simulink library "DABLib"  (R2016b)
settings: Solver=VariableStepAuto  StartTime=0.0  StopTime=10.0  RelTol=1e-3
undefined symbols (not defined in the file or in its folder): ln, sgn
libraries: DABLib x53, simulink_extras x2, simulink x1
(part 2 of 3)

== system DABLib/DABLibUtil/Medium evaporation fault f7 ==
  note: try from 0.3
  note: Fault  7
      | Medium evaporation or
      | critical pressure fault
  T[C] : Inport
  f7<0,1> : Inport  Port=2
  " " : Fcn  Expr=u(1)+200*u(4)+u(2)*u(3)*100
  Fault range <0..1> : Constant  Value=1.0
  "Fault streght saturation 0..100% " : Saturate  UpperLimit=1  LowerLimit=0
  "Fault threshold " : Constant  Value=0
  Mux4 : Mux
  Relational Operator1 : RelationalOperator  Operator=>  RndMeth=Nearest  InputSameDT=on
  Temperature range 0..300C : Saturate  UpperLimit=300  LowerLimit=0
  "Temperature range limiter 0..200C " : Saturate  UpperLimit=200  LowerLimit=0
  Tf[C] : Outport
  wires:
  " "/1 -> Temperature range 0..300C/1
  Relational Operator1/1 -> Mux4/4
  Mux4/1 -> " "/1
  "Fault streght saturation 0..100% "/1 -> Mux4/3, Relational Operator1/1
  "Fault threshold "/1 -> Relational Operator1/2
  Temperature range 0..300C/1 -> Tf[C]/1
  "Temperature range limiter 0..200C "/1 -> Mux4/1
  T[C]/1 -> "Temperature range limiter 0..200C "/1
  Fault range <0..1>/1 -> Mux4/2
  f7<0,1>/1 -> "Fault streght saturation 0..100% "/1

== system DABLib/DABLibUtil/NFSel ==
  f : Inport
  Constant4 : Constant  Value=FSel
  Constant5 : Constant  Value=0
  Demux : Demux  Outputs=19
  Multiport Switch : MultiPortSwitch  Inputs=20  SaturateOnIntegerOverflow=on  InputSameDT=on
  f(i) : Outport  InitialOutput=0
  wires:
  Demux/1 -> Multiport Switch/2
  Demux/2 -> Multiport Switch/3
  Demux/3 -> Multiport Switch/4
  Demux/4 -> Multiport Switch/5
  Demux/5 -> Multiport Switch/6
  Demux/6 -> Multiport Switch/7
  Demux/7 -> Multiport Switch/8
  Demux/8 -> Multiport Switch/9
  Demux/9 -> Multiport Switch/10
  Demux/10 -> Multiport Switch/11
  Demux/11 -> Multiport Switch/12
  Demux/12 -> Multiport Switch/13
  Demux/13 -> Multiport Switch/14
  Demux/14 -> Multiport Switch/15
  Demux/15 -> Multiport Switch/16
  Demux/16 -> Multiport Switch/17
  Demux/17 -> Multiport Switch/18
  Demux/18 -> Multiport Switch/19
  Demux/19 -> Multiport Switch/20
  f/1 -> Demux/1
  Constant4/1 -> Multiport Switch/1
  Multiport Switch/1 -> f(i)/1
  Constant5/1 -> Multiport Switch/21

== system DABLib/DABLibUtil/Positioner pressure supply fault f16 ==
  note: Fault  f16 entry
      | Positioner supply pressure fault
  Pz[Pa] : Inport
  f16 <0..1> : Inport  Port=2
  " " : Fcn  Expr=u(1)*(1-u(2)*u(3))
  Fault range in [%] <0..1> : Constant  Value=1.0
  "Fault streght saturation " : Saturate  UpperLimit=1.0  LowerLimit=0
  Mux4 : Mux  Inputs=3
  Pzf[Pa] : Outport
  wires:
  Mux4/1 -> " "/1
  Pz[Pa]/1 -> Mux4/1
  f16 <0..1>/1 -> "Fault streght saturation "/1
  " "/1 -> Pzf[Pa]/1
  "Fault streght saturation "/1 -> Mux4/3
  Fault range in [%] <0..1>/1 -> Mux4/2

== system DABLib/DABLibUtil/Tranducer ==
  X[PU] : Inport
  EN : Inport  Port=2
  fs<-1,1> : Inport  Port=3
  ADist : DABLib/DABLibUtil/ADist  Sine=on  BLWN=on  Seed=Sd  ST=0.0025
  Saturation6 : Saturate  UpperLimit=1  LowerLimit=0
  Scalling factor ScFac=1 : Gain  Gain=1/ScFact  SaturateOnIntegerOverflow=on  OutDataTypeStr=Inherit: Same as input  ParamDataTypeStr=Inherit: Same as input
  "Sensor fault " : Subsystem
  X[0...1] : Outport  InitialOutput=0
  wires:
  X[PU]/1 -> Scalling factor ScFac=1/1
  Scalling factor ScFac=1/1 -> "Sensor fault "/1(X[%])
  ADist/1 -> Saturation6/1
  Saturation6/1 -> X[0...1]/1
  EN/1 -> ADist/2
  "Sensor fault "/1(Xf[%]) -> ADist/1
  fs<-1,1>/1 -> "Sensor fault "/2(fs<-1,1>])

== system DABLib/DABLibUtil/Treshold2 ==
  In : Inport
  Constant5 : Constant  Value=TH
  Relational Operator1 : RelationalOperator  RndMeth=Nearest  InputSameDT=on
  Out : Outport  InitialOutput=0
  wires:
  Constant5/1 -> Relational Operator1/2
  In/1 -> Relational Operator1/1
  Relational Operator1/1 -> Out/1

== system DABLib/DGen/F_CV3 ==
  P6 : Constant  Value=c
  Signal Generator : SignalGenerator  Amplitude=A  Frequency=f
  suma : Sum  SaturateOnIntegerOverflow=on  InputSameDT=on  OutDataTypeStr=Inherit: Same as first input
  y : Outport  InitialOutput=0
  wires:
  suma/1 -> y/1
  P6/1 -> suma/2
  Signal Generator/1 -> suma/1

== system DABLib/DGen/F_CV4 ==
  P6 : Constant  Value=c
  Signal Generator : SignalGenerator  Amplitude=A  Frequency=f
  suma : Sum  SaturateOnIntegerOverflow=on  InputSameDT=on  OutDataTypeStr=Inherit: Same as first input
  y : Outport  InitialOutput=0
  wires:
  suma/1 -> y/1
  P6/1 -> suma/2
  Signal Generator/1 -> suma/1

== system DABLib/DGen/F_CV5 ==
  P6 : Constant  Value=c
  Signal Generator : SignalGenerator  Amplitude=A  Frequency=f
  suma : Sum  SaturateOnIntegerOverflow=on  InputSameDT=on  OutDataTypeStr=Inherit: Same as first input
  y : Outport  InitialOutput=0
  wires:
  suma/1 -> y/1
  P6/1 -> suma/2
  Signal Generator/1 -> suma/1

== system DABLib/DGen/Fault Selector ==
  f : Inport
  Constant3 : Constant  Value=[1 2 3 4 5 6 7 8 9 10 11 12 13 14 15 16 17 18 19]
  Constant4 : Constant  Value=FSel
  Constant6 : Constant  Value=0
  Demux : Demux  Outputs=19
  Multiport Switch : MultiPortSwitch  Inputs=20  SaturateOnIntegerOverflow=on  InputSameDT=on
  Product : Product  SaturateOnIntegerOverflow=on  RndMeth=Zero  InputSameDT=on  OutDataTypeStr=Inherit: Same as first input
  Relational Operator : RelationalOperator  Operator===  RndMeth=Nearest  InputSameDT=on
  f(i) : Outport  InitialOutput=0
  max(f) : Outport  Port=2  InitialOutput=0
  wires:
  Relational Operator/1 -> Product/1
  Constant3/1 -> Relational Operator/1
  f/1 -> Product/2
  Demux/2 -> Multiport Switch/3
  Demux/1 -> Multiport Switch/2
  Constant4/1 -> Relational Operator/2, Multiport Switch/1
  Product/1 -> f(i)/1, Demux/1
  Constant6/1 -> Multiport Switch/21
  Multiport Switch/1 -> max(f)/1
  Demux/19 -> Multiport Switch/20
  Demux/18 -> Multiport Switch/19
  Demux/17 -> Multiport Switch/18
  Demux/16 -> Multiport Switch/17
  Demux/15 -> Multiport Switch/16
  Demux/14 -> Multiport Switch/15
  Demux/13 -> Multiport Switch/14
  Demux/12 -> Multiport Switch/13
  Demux/11 -> Multiport Switch/12
  Demux/10 -> Multiport Switch/11
  Demux/9 -> Multiport Switch/10
  Demux/8 -> Multiport Switch/9
  Demux/7 -> Multiport Switch/8
  Demux/6 -> Multiport Switch/7
  Demux/5 -> Multiport Switch/6
  Demux/4 -> Multiport Switch/5
  Demux/3 -> Multiport Switch/4

== system DABLib/FGen/Ramp ==
  Clock : Clock
  Constant : Constant  Value=start
  Constant1 : Constant  Value=X0
  Product : Product  SaturateOnIntegerOverflow=on  RndMeth=Zero  InputSameDT=on  OutDataTypeStr=Inherit: Same as first input
  Step : Step  Time=start  After=slope
  Sum : Sum  Inputs=+-  SaturateOnIntegerOverflow=on  InputSameDT=on  OutDataTypeStr=Inherit: Same as first input
  Sum1 : Sum  SaturateOnIntegerOverflow=on  InputSameDT=on  OutDataTypeStr=Inherit: Same as first input
  out1 : Outport
  wires:
  Sum/1 -> Product/2
  Constant/1 -> Sum/2
  Clock/1 -> Sum/1
  Step/1 -> Product/1
  Product/1 -> Sum1/1
  Constant1/1 -> Sum1/2
  Sum1/1 -> out1/1

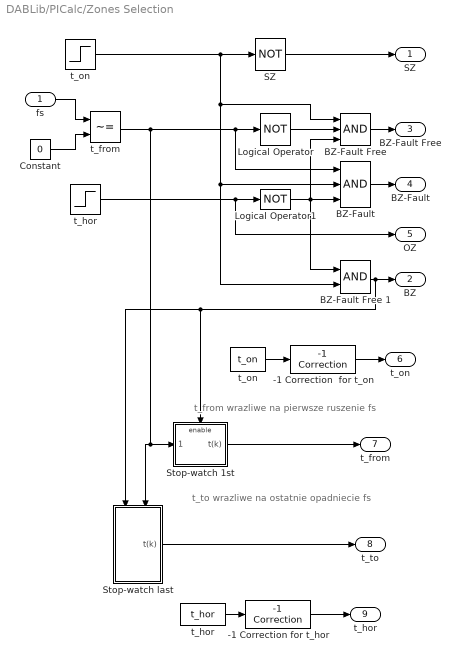
== system DABLib/PICalc/Zones Selection ==
  note: t_from wrazliwe na pierwsze ruszenie fs
  note: t_to wrazliwe na ostatnie opadniecie fs
  fs : Inport
  -1 Correction  for t_on : DABLib/DABLibUtil/-1 Correction
  -1 Correction for t_hor : DABLib/DABLibUtil/-1 Correction
  "BZ-Fault  " : Logic  Inputs=3
  "BZ-Fault Free " : Logic  Inputs=3
  BZ-Fault Free 1 : Logic
  Constant : Constant  Value=0
  Logical Operator : Logic  Operator=NOT  Inputs=1
  Logical Operator1 : Logic  Operator=NOT  Inputs=1
  "SZ " : Logic  Operator=NOT  Inputs=1
  Stop-watch 1st : Subsystem
  Stop-watch last : Subsystem
  "t_from " : RelationalOperator  Operator=~=  RndMeth=Nearest  InputSameDT=on
  "t_hor " : Step  Time=t_hor
  "t_hor   " : Constant  Value=t_hor
  "t_on " : Step  Time=t_on
  "t_on  " : Constant  Value=t_on
  SZ : Outport  InitialOutput=0
  BZ : Outport  Port=2  InitialOutput=0
  BZ-Fault Free : Outport  Port=3  InitialOutput=0
  BZ-Fault : Outport  Port=4  InitialOutput=0
  OZ : Outport  Port=5  InitialOutput=0
  t_on : Outport  Port=6  InitialOutput=0
  t_from : Outport  Port=7  InitialOutput=0
  t_to : Outport  Port=8  InitialOutput=0
  "t_hor  " : Outport  Port=9  InitialOutput=0
  wires:
  "SZ "/1 -> SZ/1
  "t_on "/1 -> "SZ "/1, "BZ-Fault Free "/1, "BZ-Fault  "/2, BZ-Fault Free 1/2
  Constant/1 -> "t_from "/2
  fs/1 -> "t_from "/1
  "t_from "/1 -> Logical Operator/1, "BZ-Fault  "/1, Stop-watch 1st/1(TR st), Stop-watch last/Trigger
  Logical Operator/1 -> "BZ-Fault Free "/2
  Logical Operator1/1 -> "BZ-Fault  "/3, "BZ-Fault Free "/3, BZ-Fault Free 1/1
  "BZ-Fault  "/1 -> BZ-Fault/1
  "BZ-Fault Free "/1 -> BZ-Fault Free/1
  "t_hor "/1 -> Logical Operator1/1, OZ/1
  BZ-Fault Free 1/1 -> BZ/1, Stop-watch 1st/Enable, Stop-watch last/Enable
  -1 Correction  for t_on/1 -> t_on/1
  -1 Correction for t_hor/1 -> "t_hor  "/1
  "t_on  "/1 -> -1 Correction  for t_on/1
  "t_hor   "/1 -> -1 Correction for t_hor/1
  Stop-watch last/1(t(k)) -> t_to/1
  Stop-watch 1st/1(t(k)) -> t_from/1

== system DABLib/PICalc/subsystem ==
  t_on : Inport
  t_hor : Inport  Port=2
  CID : Inport  Port=3
  Enable : EnablePort
  0 Proof Division with -1 correction : DABLib/DABLibUtil/0 Proof Division with -1 correction
  "0, t-t1>0, t2 or 0" : DABLib/DABLibUtil/0, t-t1>0, t2 or 0
  t_mi_CID : Integrator
  r_mi : Outport  InitialOutput=0
  wires:
  t_hor/1 -> "0, t-t1>0, t2 or 0"/1
  0 Proof Division with -1 correction/1 -> r_mi/1
  t_on/1 -> "0, t-t1>0, t2 or 0"/2
  "0, t-t1>0, t2 or 0"/1 -> 0 Proof Division with -1 correction/1
  CID/1 -> t_mi_CID/1
  t_mi_CID/1 -> 0 Proof Division with -1 correction/2

== system DABLib/ProcessBlk/ProcAct ==
  CV : Inport
  P1[Pa] : Inport  Port=2
  P2[Pa] : Inport  Port=3
  T1[C] : Inport  Port=4
  Pz[Pa] : Inport  Port=5
  f : Inport  Port=6
  CoreAct : DABLib/DABLibUtil/CoreAct
  Demux : Demux  Outputs=19
  Terminator{2..6} (5 alike) : Terminator
  Fv[t/h] : Outport  InitialOutput=0
  Pz' : Outport  Port=2  InitialOutput=0
  CVI' : Outport  Port=3  InitialOutput=0
  Ps' : Outport  Port=4  InitialOutput=0
  X' : Outport  Port=5  InitialOutput=0
  wires:
  Demux/19 -> Terminator2/1
  CoreAct/2 -> X'/1
  CoreAct/3 -> Pz'/1
  CoreAct/4 -> CVI'/1
  Demux/1 -> CoreAct/6
  f/1 -> Demux/1
  Demux/2 -> CoreAct/7
  Demux/3 -> CoreAct/8
  Demux/4 -> CoreAct/9
  Demux/5 -> CoreAct/10
  Demux/6 -> CoreAct/11
  Demux/18 -> Terminator3/1
  Demux/16 -> Terminator5/1
  CoreAct/1 -> Fv[t/h]/1
  CoreAct/5 -> Ps'/1
  CV/1 -> CoreAct/5
  T1[C]/1 -> CoreAct/3
  Pz[Pa]/1 -> CoreAct/4
  P2[Pa]/1 -> CoreAct/2
  P1[Pa]/1 -> CoreAct/1
  Demux/17 -> Terminator4/1
  Demux/8 -> CoreAct/12
  Demux/9 -> CoreAct/13
  Demux/10 -> CoreAct/14
  Demux/11 -> CoreAct/15
  Demux/12 -> CoreAct/16
  Demux/13 -> CoreAct/17
  Demux/14 -> CoreAct/18
  Demux/15 -> CoreAct/19
  Demux/7 -> Terminator6/1

== system DABLib/ProcessBlk/ProcBV ==
  Xb : Inport
  P1[Pa] : Inport  Port=2
  P2[Pa] : Inport  Port=3
  T1[C] : Inport  Port=4
  ByVal : DABLib/DABLibUtil/ByVal
  Fv3[m3/h] : Outport  InitialOutput=0
  wires:
  ByVal/1 -> Fv3[m3/h]/1
  Xb/1 -> ByVal/1
  P1[Pa]/1 -> ByVal/2
  P2[Pa]/1 -> ByVal/3
  T1[C]/1 -> ByVal/4

== system DABLib/ProcessBlk/ProcTran ==
  in : Inport
  f : Inport  Port=2
  Constant4 : Constant  Value=FSel
  Constant5 : Constant  Value=0
  Demux : Demux  Outputs=19
  Multiport Switch : MultiPortSwitch  Inputs=20  SaturateOnIntegerOverflow=on  InputSameDT=on
  Sine1 : Constant  Value=EN
  Tranducer : DABLib/DABLibUtil/Tranducer  ScFact=ScFact  Sd=Sd
  out : Outport  InitialOutput=0
  wires:
  in/1 -> Tranducer/1
  Sine1/1 -> Tranducer/2
  Demux/1 -> Multiport Switch/2
  Demux/2 -> Multiport Switch/3
  Demux/3 -> Multiport Switch/4
  Demux/4 -> Multiport Switch/5
  Demux/5 -> Multiport Switch/6
  Demux/6 -> Multiport Switch/7
  Demux/7 -> Multiport Switch/8
  Demux/8 -> Multiport Switch/9
  Demux/9 -> Multiport Switch/10
  Demux/10 -> Multiport Switch/11
  Demux/11 -> Multiport Switch/12
  Demux/12 -> Multiport Switch/13
  Demux/13 -> Multiport Switch/14
  Demux/14 -> Multiport Switch/15
  Demux/15 -> Multiport Switch/16
  Demux/16 -> Multiport Switch/17
  Demux/17 -> Multiport Switch/18
  Demux/18 -> Multiport Switch/19
  Demux/19 -> Multiport Switch/20
  f/1 -> Demux/1
  Constant4/1 -> Multiport Switch/1
  Constant5/1 -> Multiport Switch/21
  Tranducer/1 -> out/1
  Multiport Switch/1 -> Tranducer/3

== system DABLib/ProcessBlk/Proc_f16 ==
  Pz[Pa] : Inport
  f : Inport  Port=2
  NFSel : DABLib/DABLibUtil/NFSel  FSel=f16 - Positioner supply pressure drop
  Positioner pressure supply fault f16 : DABLib/DABLibUtil/Positioner pressure  supply fault f16
  Pzf[Pa] : Outport  InitialOutput=0
  wires:
  f/1 -> NFSel/1
  NFSel/1 -> Positioner pressure supply fault f16/2
  Positioner pressure supply fault f16/1 -> Pzf[Pa]/1
  Pz[Pa]/1 -> Positioner pressure supply fault f16/1

== system DABLib/ProcessBlk/Proc_f18 ==
  f : Inport
  Bypass valve opened or bypass valve leaky f18 : DABLib/DABLibUtil/Bypass valve opened  or bypass valve leaky  f18
  NFSel : DABLib/DABLibUtil/NFSel  FSel=f18 - Fully or partly opened bypass valves
  Xb[%] : Outport  InitialOutput=0
  wires:
  Bypass valve opened or bypass valve leaky f18/1 -> Xb[%]/1
  f/1 -> NFSel/1
  NFSel/1 -> Bypass valve opened or bypass valve leaky f18/1

== system DABLib/ProcessBlk/Proc_f7 ==
  T1[C] : Inport
  f : Inport  Port=2
  "Medium evaporation fault f7 " : DABLib/DABLibUtil/Medium evaporation fault f7
  NFSel : DABLib/DABLibUtil/NFSel  FSel=f7 - Medium evaporation or critical flow
  T1f[C] : Outport  InitialOutput=0
  wires:
  T1[C]/1 -> "Medium evaporation fault f7 "/1
  "Medium evaporation fault f7 "/1 -> T1f[C]/1
  NFSel/1 -> "Medium evaporation fault f7 "/2
  f/1 -> NFSel/1

== system DABLib/DABLibUtil/CoreAct/  E//P transducer ==
  note: E/P transducer
  CVI : Inport
  f12<-1,1> : Inport  Port=2
  E/P look-up table : Lookup  InputValues=[-1.00, -0.94, -0.54, 0.46, 0.86, 1.00]  Table=[-0.55 -0.55 -0.02, 0.02, 1.00 1.00]  SaturateOnIntegerOverflow=on
  E/P transducer saturation -1..+1 : Saturate  UpperLimit=1.0  LowerLimit=-1.0
  Electro-pneumatic transducer  fault f12 : Subsystem
  Input saturation -1..+1 : Saturate  UpperLimit=1.0  LowerLimit=-1.0
  CVP[%] : Outport
  wires:
  E/P transducer saturation -1..+1/1 -> CVP[%]/1
  Electro-pneumatic transducer  fault f12/1(If[%]) -> E/P transducer saturation -1..+1/1
  E/P look-up table/1 -> Electro-pneumatic transducer  fault f12/1(I[%])
  CVI/1 -> Input saturation -1..+1/1
  f12<-1,1>/1 -> Electro-pneumatic transducer  fault f12/2(f12<-1,1>])
  Input saturation -1..+1/1 -> E/P look-up table/1

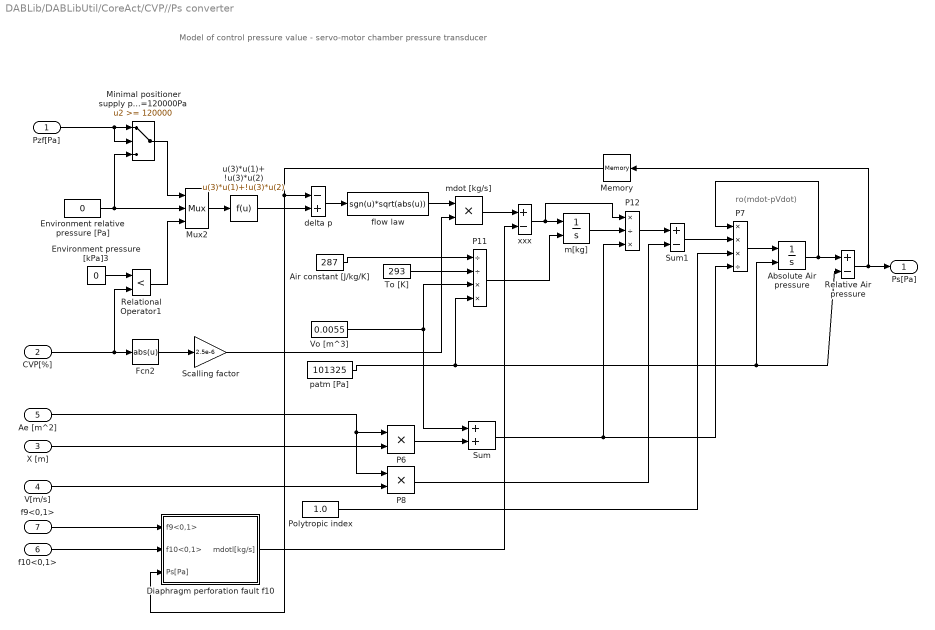
== system DABLib/DABLibUtil/CoreAct/CVP//Ps converter ==
  note: ro(mdot-pVdot)
  note: Model of control pressure value - servo-motor chamber pressure transducer
  Pzf[Pa] : Inport
  CVP[%] : Inport  Port=2
  X [m] : Inport  Port=3
  V[m/s] : Inport  Port=4
  Ae [m^2] : Inport  Port=5
  f10<0,1> : Inport  Port=6
  f9<0,1> : Inport  Port=7
  Absolute Air pressure : Integrator  InitialConditionSource=external  LimitOutput=on  UpperSaturationLimit=700000  LowerSaturationLimit=0
  Air constant [J/kg/K] : Constant  Value=287
  Diaphragm perforation fault f10 : Subsystem
  Environment pressure [kPa]3 : Constant  Value=0
  Environment relative pressure [Pa] : Constant  Value=0
  Fcn2 : Fcn  Expr=abs(u)
  Memory : Memory
  Minimal positioner supply pressure =120000Pa : Switch  Threshold=120000  SaturateOnIntegerOverflow=on  InputSameDT=on
  Mux2 : Mux  Inputs=3
  P11 : Product  Inputs=//**  SaturateOnIntegerOverflow=on  RndMeth=Zero  InputSameDT=on  OutDataTypeStr=Inherit: Same as first input
  P12 : Product  Inputs=*/*  SaturateOnIntegerOverflow=on  RndMeth=Zero  InputSameDT=on  OutDataTypeStr=Inherit: Same as first input
  P6 : Product  SaturateOnIntegerOverflow=on  RndMeth=Zero  InputSameDT=on  OutDataTypeStr=Inherit: Same as first input
  P7 : Product  Inputs=***/  SaturateOnIntegerOverflow=on  RndMeth=Zero  InputSameDT=on  OutDataTypeStr=Inherit: Same as first input
  P8 : Product  SaturateOnIntegerOverflow=on  RndMeth=Zero  InputSameDT=on  OutDataTypeStr=Inherit: Same as first input
  Polytropic index : Constant  Value=1.0
  Relational Operator1 : RelationalOperator  Operator=<  RndMeth=Nearest  InputSameDT=on
  Relative Air pressure : Sum  Inputs=+-  SaturateOnIntegerOverflow=on  InputSameDT=on  OutDataTypeStr=Inherit: Same as first input
  Scalling factor : Gain  Gain=2.5e-6  SaturateOnIntegerOverflow=on  OutDataTypeStr=Inherit: Same as input  ParamDataTypeStr=Inherit: Same as input
  Sum : Sum  SaturateOnIntegerOverflow=on  InputSameDT=on  OutDataTypeStr=Inherit: Same as first input
  Sum1 : Sum  Inputs=+-  SaturateOnIntegerOverflow=on  InputSameDT=on  OutDataTypeStr=Inherit: Same as first input
  To [K] : Constant  Value=293
  Vo [m^3] : Constant  Value=0.0055
  "delta p " : Sum  Inputs=-+  SaturateOnIntegerOverflow=on  InputSameDT=on  OutDataTypeStr=Inherit: Same as first input
  flow law : Fcn  Expr=sgn(u)*sqrt(abs(u))
  "m[kg] " : Integrator  InitialConditionSource=external  InitialCondition=2.41e-3  LimitOutput=on  UpperSaturationLimit=0.1  LowerSaturationLimit=0
  mdot [kg/s] : Product  SaturateOnIntegerOverflow=on  RndMeth=Zero  InputSameDT=on  OutDataTypeStr=Inherit: Same as first input
  patm [Pa] : Constant  Value=101325
  u(3)*u(1)+ !u(3)*u(2) : Fcn  Expr=u(3)*u(1)+!u(3)*u(2)
  xxx : Sum  Inputs=+-  SaturateOnIntegerOverflow=on  InputSameDT=on  OutDataTypeStr=Inherit: Same as first input
  Ps[Pa] : Outport
  wires:
  xxx/1 -> P12/1, "m[kg] "/1
  P8/1 -> Sum1/2
  Sum1/1 -> P7/2
  P12/1 -> Sum1/1
  "m[kg] "/1 -> P12/2
  Scalling factor/1 -> mdot [kg/s]/2
  Vo [m^3]/1 -> Sum/1, P11/3
  patm [Pa]/1 -> Absolute Air pressure/2, Relative Air pressure/2, P11/4
  To [K]/1 -> P11/2
  Air constant [J/kg/K]/1 -> P11/1
  Memory/1 -> "delta p "/1, Diaphragm perforation fault f10/3(Ps[Pa])
  mdot [kg/s]/1 -> xxx/1
  Diaphragm perforation fault f10/1(mdotl[kg/s]) -> xxx/2
  Polytropic index/1 -> P7/3
  V[m/s]/1 -> P8/2
  X [m]/1 -> P6/2
  Ae [m^2]/1 -> P8/1, P6/1
  Sum/1 -> P7/4, P12/3
  P6/1 -> Sum/2
  Relative Air pressure/1 -> Memory/1, Ps[Pa]/1
  Absolute Air pressure/1 -> P7/1, Relative Air pressure/1
  P7/1 -> Absolute Air pressure/1
  P11/1 -> "m[kg] "/2
  flow law/1 -> mdot [kg/s]/1
  "delta p "/1 -> flow law/1
  f9<0,1>/1 -> Diaphragm perforation fault f10/1(f9<0,1>)
  f10<0,1>/1 -> Diaphragm perforation fault f10/2(f10<0,1>)
  Environment relative pressure [Pa]/1 -> Minimal positioner supply pressure =120000Pa/3, Mux2/2
  Minimal positioner supply pressure =120000Pa/1 -> Mux2/1
  Pzf[Pa]/1 -> Minimal positioner supply pressure =120000Pa/1, Minimal positioner supply pressure =120000Pa/2
  Fcn2/1 -> Scalling factor/1
  u(3)*u(1)+ !u(3)*u(2)/1 -> "delta p "/2
  CVP[%]/1 -> Relational Operator1/2, Fcn2/1
  Environment pressure [kPa]3/1 -> Relational Operator1/1
  Relational Operator1/1 -> Mux2/3
  Mux2/1 -> u(3)*u(1)+ !u(3)*u(2)/1

== system DABLib/DABLibUtil/CoreAct/Diaphragm perforation fault f10 ==
  note: Fault  f10
      | Servomotor's diaphragm perforation fault
  Ae[m^2] : Inport
  f10 <0..1> : Inport  Port=2
  " " : Fcn  Expr=u(1)*(1-u(2)*u(3))
  Fault range in [%] <0..1> : Constant  Value=1.0
  "Fault streght saturation " : Saturate  UpperLimit=1.0  LowerLimit=0
  Mux4 : Mux  Inputs=3
  Aef[m^2] : Outport
  wires:
  " "/1 -> Aef[m^2]/1
  Ae[m^2]/1 -> Mux4/1
  Mux4/1 -> " "/1
  Fault range in [%] <0..1>/1 -> Mux4/2
  "Fault streght saturation "/1 -> Mux4/3
  f10 <0..1>/1 -> "Fault streght saturation "/1

== system DABLib/DABLibUtil/CoreAct/External leakage leaky bushing, covers, terminals fault  f5 ==
  note: Fault  f5
      | External leakage fault
  Fv[t/h] : Inport
  f5<0,1>] : Inport  Port=2
  " " : Fcn  Expr=u(1)*(1-u(2)*u(3))
  Fault range in [%] <0..1> : Constant  Value=0.05
  "Fault streght saturation 0..100% " : Saturate  UpperLimit=1.0  LowerLimit=0.0
  Mux4 : Mux  Inputs=3
  Fv(f5)[t/h] : Outport
  wires:
  Fault range in [%] <0..1>/1 -> Mux4/2
  "Fault streght saturation 0..100% "/1 -> Mux4/3
  " "/1 -> Fv(f5)[t/h]/1
  f5<0,1>]/1 -> "Fault streght saturation 0..100% "/1
  Fv[t/h]/1 -> Mux4/1
  Mux4/1 -> " "/1

== system DABLib/DABLibUtil/CoreAct/II order lag filter ==
  note: II order lag filter
  u[%] : Inport
  I order lag : TransferFcn  Denominator=[0.30 1]
  I order lag1 : TransferFcn  Denominator=[0.30 1]
  hardware saturation 0 .. 1.024 : Saturate  UpperLimit=1.024  LowerLimit=0
  "numerical saturation -128..127 " : Saturate  UpperLimit=127  LowerLimit=-128
  "numerical saturation -128..127 " : Saturate  UpperLimit=127  LowerLimit=-128
  y[%] : Outport
  wires:
  hardware saturation 0 .. 1.024/1 -> I order lag/1
  u[%]/1 -> hardware saturation 0 .. 1.024/1
  "numerical saturation -128..127 "/1 -> y[%]/1
  I order lag1/1 -> "numerical saturation -128..127 "/1
  "numerical saturation -128..127 "/1 -> I order lag1/1
  I order lag/1 -> "numerical saturation -128..127 "/1

== system DABLib/DABLibUtil/CoreAct/P-controller ==
  note: P controller
  SP+ : Inport
  PV- : Inport  Port=2
  " " : Constant
  "  " : Gain  Gain=0.5  SaturateOnIntegerOverflow=on  OutDataTypeStr=Inherit: Same as input  ParamDataTypeStr=Inherit: Same as input
  Booster Gain factor : Gain  SaturateOnIntegerOverflow=on  OutDataTypeStr=Inherit: Same as input  ParamDataTypeStr=Inherit: Same as input
  "Booster saturation -128 .. 127 " : Saturate  UpperLimit=1.0  LowerLimit=-1.0
  Controller Gain factor nominal kp =100 : Gain  Gain=100  SaturateOnIntegerOverflow=on  OutDataTypeStr=Inherit: Same as input  ParamDataTypeStr=Inherit: Same as input
  "Controller saturation -128 .. 127 " : Saturate  UpperLimit=127  LowerLimit=-128
  Sum2 : Sum  Inputs=+-  SaturateOnIntegerOverflow=on  InputSameDT=on  OutDataTypeStr=Inherit: Same as first input
  Sum3 : Sum  SaturateOnIntegerOverflow=on  InputSameDT=on  OutDataTypeStr=Inherit: Same as first input
  Zero-Order Hold : ZeroOrderHold  SampleTime=0.035
  CVI[0,1] : Outport
  CVI[-1,1] : Outport  Port=2
  wires:
  "  "/1 -> CVI[0,1]/1
  Sum3/1 -> "  "/1
  Zero-Order Hold/1 -> Sum3/1, CVI[-1,1]/1
  " "/1 -> Sum3/2
  "Booster saturation -128 .. 127 "/1 -> Zero-Order Hold/1
  Controller Gain factor nominal kp =100/1 -> "Controller saturation -128 .. 127 "/1
  "Controller saturation -128 .. 127 "/1 -> Booster Gain factor/1
  Booster Gain factor/1 -> "Booster saturation -128 .. 127 "/1
  SP+/1 -> Sum2/1
  PV-/1 -> Sum2/2
  Sum2/1 -> Controller Gain factor nominal kp =100/1

== system DABLib/DABLibUtil/CoreAct/Positioner feedback ==
  note: -50..+50%
  note: Positioner feedback
  X[m] : Inport
  f15<0,1> : Inport  Port=2
  " " : Fcn  Description=Potentiometer angle  Expr=asin(u)*180/3.1415926
  " 2" : Product  Inputs=/*  SaturateOnIntegerOverflow=on  RndMeth=Zero  InputSameDT=on  OutDataTypeStr=Inherit: Same as first input
  Gain PV 1=100[%] : Gain  SaturateOnIntegerOverflow=on  OutDataTypeStr=Inherit: Same as input  ParamDataTypeStr=Inherit: Same as input
  Nominal valve plug travel in [m] : Constant  Value=0.0381
  Offset 50[%] : Constant  Value=0.5
  Positioner feedback fault f15 : Subsystem
  "Scalling factor 100%=60.00deg " : Gain  Gain=1/60  SaturateOnIntegerOverflow=on  OutDataTypeStr=Inherit: Same as input  ParamDataTypeStr=Inherit: Same as input
  Sum2 : Sum  SaturateOnIntegerOverflow=on  InputSameDT=on  OutDataTypeStr=Inherit: Same as first input
  Sum3 : Sum  Inputs=+-  SaturateOnIntegerOverflow=on  InputSameDT=on  OutDataTypeStr=Inherit: Same as first input
  WUT Backlash : Subsystem
  Xo/2[m] Nominal stroke/2 Initlial positioner adjustment : Constant  Value=0.01905
  hardware bumps -0.02 .. 0.05 : Saturate  UpperLimit=0.05  LowerLimit=-0.01
  l[m] Lever length : Constant  Value=0.0381
  look-up table Set as linear : Lookup  InputValues=[-2.00, 2.00]  Table=[-2.00, 2.00]  SaturateOnIntegerOverflow=on
  numerical saturation -1..2 : Saturate  UpperLimit=2  LowerLimit=-2
  "numerical saturation -128..127 " : Saturate  UpperLimit=127  LowerLimit=-128
  PV[%] : Outport
  wires:
  hardware bumps -0.02 .. 0.05/1 -> WUT Backlash/1(signal)
  Sum3/1 -> " 2"/2
  " "/1 -> "Scalling factor 100%=60.00deg "/1
  Gain PV 1=100[%]/1 -> "numerical saturation -128..127 "/1
  Offset 50[%]/1 -> Sum2/2
  "Scalling factor 100%=60.00deg "/1 -> Sum2/1
  Xo/2[m] Nominal stroke/2 Initlial positioner adjustment/1 -> Sum3/2
  " 2"/1 -> " "/1
  WUT Backlash/1(output) -> Sum3/1
  Positioner feedback fault f15/1(Df[m]) -> WUT Backlash/2(dead band)
  Nominal valve plug travel in [m]/1 -> Positioner feedback fault f15/1(Xn[m])
  f15<0,1>/1 -> Positioner feedback fault f15/2(f15<0,1>)
  X[m]/1 -> hardware bumps -0.02 .. 0.05/1
  l[m] Lever length/1 -> " 2"/1
  Sum2/1 -> numerical saturation -1..2/1
  numerical saturation -1..2/1 -> look-up table Set as linear/1
  "numerical saturation -128..127 "/1 -> PV[%]/1
  look-up table Set as linear/1 -> Gain PV 1=100[%]/1

== system DABLib/DABLibUtil/CoreAct/Pressure sensor fault f14 ==
  note: Fault  f14 entry
      | Pressure sensor fault
  Ps[Pa] : Inport
  f14<-1,1>] : Inport  Port=2
  " " : Fcn  Expr=u(1)*(1-u(2)*u(3))
  Fault range <0..1> : Constant  Value=1.00
  "Fault streght saturation -1..1 " : Saturate  UpperLimit=1.0  LowerLimit=-1.0
  Mux4 : Mux  Inputs=3
  Scalling factor 1=600000[Pa] : Gain  Gain=1/1000000  SaturateOnIntegerOverflow=on  OutDataTypeStr=Inherit: Same as input  ParamDataTypeStr=Inherit: Same as input
  Sensor range 0..1 : Saturate  UpperLimit=1.00  LowerLimit=0
  "Sensor range 0..1 " : Saturate  UpperLimit=1  LowerLimit=0
  Psf[0..1] : Outport
  wires:
  Scalling factor 1=600000[Pa]/1 -> "Sensor range 0..1 "/1
  Ps[Pa]/1 -> Scalling factor 1=600000[Pa]/1
  Mux4/1 -> " "/1
  f14<-1,1>]/1 -> "Fault streght saturation -1..1 "/1
  "Fault streght saturation -1..1 "/1 -> Mux4/3
  Fault range <0..1>/1 -> Mux4/2
  "Sensor range 0..1 "/1 -> Mux4/1
  " "/1 -> Sensor range 0..1/1
  Sensor range 0..1/1 -> Psf[0..1]/1

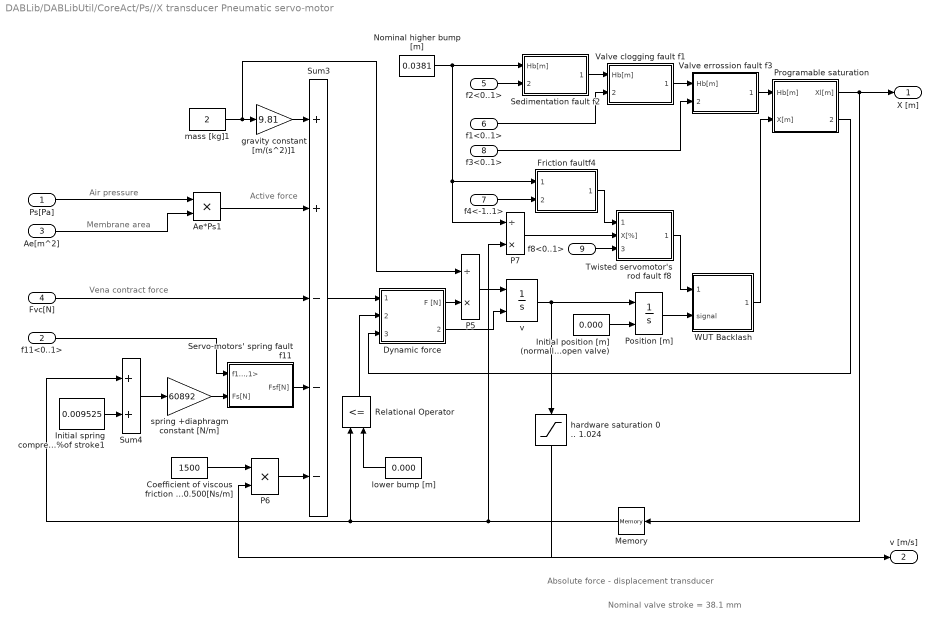
== system DABLib/DABLibUtil/CoreAct/Ps//X transducer Pneumatic servo-motor ==
  note: Nominal valve stroke = 38.1 mm
  note: Active force
  note: Membrane area
  note: Air pressure
  note: Vena contract force
  note: Absolute force - displacement transducer
  Ps[Pa] : Inport
  f11<0..1> : Inport  Port=2
  Ae[m^2] : Inport  Port=3
  Fvc[N] : Inport  Port=4
  f2<0..1> : Inport  Port=5
  f1<0..1> : Inport  Port=6
  f4<-1..1> : Inport  Port=7
  f3<0..1> : Inport  Port=8
  f8<0..1> : Inport  Port=9
  Ae*Ps1 : Product  SaturateOnIntegerOverflow=on  RndMeth=Zero  InputSameDT=on  OutDataTypeStr=Inherit: Same as first input
  Coefficient of viscous friction 20.500[Ns/m] : Constant  Value=1500
  Dynamic force : Subsystem
  Friction faultf4 : Subsystem
  Initial position [m] (normally open valve) : Constant  Value=0.000
  Initial spring compression [m] 25%of stroke1 : Constant  Value=0.009525
  Memory : Memory
  "Nominal higher bump [m] " : Constant  Value=0.0381
  P5 : Product  Inputs=/*  SaturateOnIntegerOverflow=on  RndMeth=Zero  InputSameDT=on  OutDataTypeStr=Inherit: Same as first input
  P6 : Product  Inputs=**  SaturateOnIntegerOverflow=on  RndMeth=Zero  InputSameDT=on  OutDataTypeStr=Inherit: Same as first input
  P7 : Product  Inputs=/*  SaturateOnIntegerOverflow=on  RndMeth=Zero  InputSameDT=on  OutDataTypeStr=Inherit: Same as first input
  Position [m] : Integrator  InitialConditionSource=external  LimitOutput=on  UpperSaturationLimit=0.0381*1.25  LowerSaturationLimit=-0.05*0.0381
  Programable saturation : Subsystem
  Relational Operator : RelationalOperator  Operator=<=  RndMeth=Nearest  InputSameDT=on
  Sedimentation fault f2 : Subsystem
  Servo-motors' spring fault f11 : Subsystem
  Sum3 : Sum  Inputs=++---  SaturateOnIntegerOverflow=on  InputSameDT=on  OutDataTypeStr=Inherit: Same as first input
  Sum4 : Sum  SaturateOnIntegerOverflow=on  InputSameDT=on  OutDataTypeStr=Inherit: Same as first input
  Twisted servomotor's rod fault f8 : Subsystem
  Valve clogging fault f1 : Subsystem
  Valve errossion fault f3 : Subsystem
  WUT Backlash : Subsystem
  gravity constant [m/(s^2)]1 : Gain  Gain=9.81  SaturateOnIntegerOverflow=on  OutDataTypeStr=Inherit: Same as input  ParamDataTypeStr=Inherit: Same as input
  hardware saturation 0 .. 1.024 : Saturate  UpperLimit=0.02  LowerLimit=-0.02
  "lower bump [m] " : Constant  Value=0.000
  mass [kg]1 : Constant  Value=2
  spring +diaphragm constant [N/m] : Gain  Gain=60892  SaturateOnIntegerOverflow=on  OutDataTypeStr=Inherit: Same as input  ParamDataTypeStr=Inherit: Same as input
  v : Integrator  ExternalReset=either  LowerSaturationLimit=-0.002
  X [m] : Outport  InitialOutput=0
  v [m/s] : Outport  Port=2  InitialOutput=0
  wires:
  hardware saturation 0 .. 1.024/1 -> v [m/s]/1
  Dynamic force/2(V reset) -> v/2
  Memory/1 -> P7/2, Relational Operator/1, Sum4/1
  Ae*Ps1/1 -> Sum3/2
  mass [kg]1/1 -> P5/1, gravity constant [m/(s^2)]1/1
  f11<0..1>/1 -> Servo-motors' spring fault f11/1(f11<0,1>)
  Servo-motors' spring fault f11/1(Fsf[N]) -> Sum3/4
  spring +diaphragm constant [N/m]/1 -> Servo-motors' spring fault f11/2(Fs[N])
  Sum4/1 -> spring +diaphragm constant [N/m]/1
  Fvc[N]/1 -> Sum3/3
  gravity constant [m/(s^2)]1/1 -> Sum3/1
  Initial spring compression [m] 25%of stroke1/1 -> Sum4/2
  Coefficient of viscous friction 20.500[Ns/m]/1 -> P6/1
  P6/1 -> Sum3/5
  Ps[Pa]/1 -> Ae*Ps1/1
  Ae[m^2]/1 -> Ae*Ps1/2
  Sum3/1 -> Dynamic force/1(Fd'A [N])
  Relational Operator/1 -> Dynamic force/2(X<=Lb)
  Initial position [m] (normally open valve)/1 -> Position [m]/2
  P5/1 -> v/1
  "lower bump [m] "/1 -> Relational Operator/2
  Dynamic force/1(F [N]) -> P5/2
  v/1 -> hardware saturation 0 .. 1.024/1, P6/2, Position [m]/1
  Position [m]/1 -> WUT Backlash/2(signal)
  f4<-1..1>/1 -> Friction faultf4/2(f4<-1,1>)
  Valve clogging fault f1/1(Hbf[m]) -> Valve errossion fault f3/1(Hb[m])
  Sedimentation fault f2/1(Hbf[m]) -> Valve clogging fault f1/1(Hb[m])
  f3<0..1>/1 -> Valve errossion fault f3/2(f3<0,1>)
  f2<0..1>/1 -> Sedimentation fault f2/2(f2<0,1>)
  f1<0..1>/1 -> Valve clogging fault f1/2(f1<0,1>)
  WUT Backlash/1(output) -> Programable saturation/2(X[m])
  Valve errossion fault f3/1(Hbf[m]) -> Programable saturation/1(Hb[m])
  Programable saturation/1(Xl[m]) -> Memory/1, X [m]/1
  Programable saturation/2(1 if Hb<=X) -> Dynamic force/3(X>=Hb)
  "Nominal higher bump [m] "/1 -> Sedimentation fault f2/1(Hb[m]), Friction faultf4/1(Hb[m]), P7/1
  f8<0..1>/1 -> Twisted servomotor's rod fault f8/3(f8<0,1>)
  Friction faultf4/1(Dbf[m]) -> Twisted servomotor's rod fault f8/1(Db[m])
  Twisted servomotor's rod fault f8/1(Dbf[m]) -> WUT Backlash/1(dead band)
  P7/1 -> Twisted servomotor's rod fault f8/2(X[%])

== system DABLib/DABLibUtil/CoreAct/Rod displacement sensor fault f13 ==
  note: Fault  f13
      | Rod displacement sensor fault
  X[m] : Inport
  f13<-1,1> : Inport  Port=2
  " " : Fcn  Expr=u(1)*(1+u(2)*u(3))
  Fault range <0..1> : Constant  Value=1.25
  "Fault streght saturation -100..100% " : Saturate  UpperLimit=1.0  LowerLimit=-1.0
  Feedback range -25..125% : Saturate  UpperLimit=0.0381*1.25  LowerLimit=-0.25*0.0381
  Mux4 : Mux  Inputs=3
  "Sensor range -25..125% " : Saturate  UpperLimit=0.0381*1.25  LowerLimit=-0.25*0.0381
  Sensor range 0..100% : Saturate  UpperLimit=0.0381*1.00  LowerLimit=0*0.00
  X'f[m] : Outport
  Xf[m] : Outport  Port=2
  wires:
  " "/1 -> Feedback range -25..125%/1, Sensor range 0..100%/1
  Feedback range -25..125%/1 -> Xf[m]/1
  Sensor range 0..100%/1 -> X'f[m]/1
  "Sensor range -25..125% "/1 -> Mux4/1
  X[m]/1 -> "Sensor range -25..125% "/1
  Fault range <0..1>/1 -> Mux4/2
  "Fault streght saturation -100..100% "/1 -> Mux4/3
  f13<-1,1>/1 -> "Fault streght saturation -100..100% "/1
  Mux4/1 -> " "/1

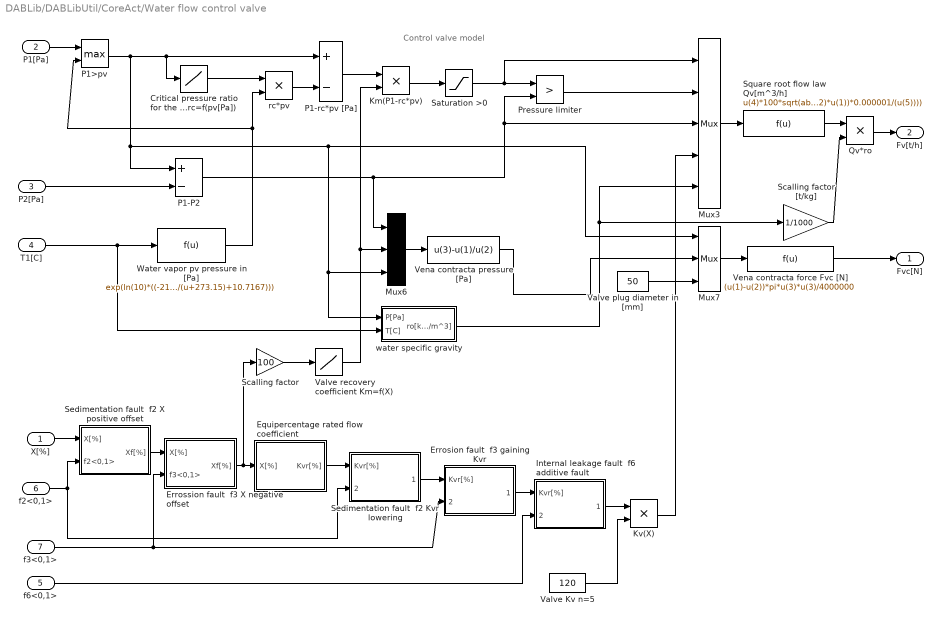
== system DABLib/DABLibUtil/CoreAct/Water flow control valve ==
  note: Control valve model
  X[%] : Inport
  P1[Pa] : Inport  Port=2
  P2[Pa] : Inport  Port=3
  T1[C] : Inport  Port=4
  f6<0,1> : Inport  Port=5
  f2<0,1> : Inport  Port=6
  f3<0,1> : Inport  Port=7
  " Valve Kv n=5" : Constant  Value=120
  "Critical pressure ratio for the water rc=f(pv[Pa]) " : Lookup  InputValues="[0  1723763 3447527 6895055 13790111 17237639 20685166]"  Table=[0.94 0.87 0.84 0.79 0.75 0.725 0.685]  SaturateOnIntegerOverflow=on
  Equipercentage rated flow coefficient : Subsystem
  "Errosion fault  f3 gaining Kvr " : Subsystem
  Errossion fault  f3 X negative offset : Subsystem
  Internal leakage fault  f6 additive fault : Subsystem
  Km(P1-rc*pv) : Product  SaturateOnIntegerOverflow=on  RndMeth=Zero  InputSameDT=on  OutDataTypeStr=Inherit: Same as first input
  Kv(X) : Product  SaturateOnIntegerOverflow=on  RndMeth=Zero  InputSameDT=on  OutDataTypeStr=Inherit: Same as first input
  Mux3 : Mux  Inputs=5
  Mux6 : Mux  Inputs=3
  Mux7 : Mux  Inputs=3
  P1-P2 : Sum  Inputs=+-  SaturateOnIntegerOverflow=on  InputSameDT=on  OutDataTypeStr=Inherit: Same as first input
  P1-rc*pv [Pa] : Sum  Inputs=+-  SaturateOnIntegerOverflow=on  InputSameDT=on  OutDataTypeStr=Inherit: Same as first input
  P1>pv : MinMax  Function=max  Inputs=2  SaturateOnIntegerOverflow=on  InputSameDT=on
  Pressure limiter : RelationalOperator  Operator=>  RndMeth=Nearest  InputSameDT=on
  Qv*ro : Product  SaturateOnIntegerOverflow=on  RndMeth=Zero  InputSameDT=on  OutDataTypeStr=Inherit: Same as first input
  Saturation >0 : Saturate  UpperLimit=inf  LowerLimit=0
  Scalling factor : Gain  Gain=100  SaturateOnIntegerOverflow=on  OutDataTypeStr=Inherit: Same as input  ParamDataTypeStr=Inherit: Same as input
  Scalling factor [t/kg] : Gain  Gain=1/1000  SaturateOnIntegerOverflow=on  OutDataTypeStr=Inherit: Same as input  ParamDataTypeStr=Inherit: Same as input
  Sedimentation fault  f2 Kvr lowering : Subsystem
  Sedimentation fault  f2 X positive offset : Subsystem
  Square root flow law Qv[m^3/h] : Fcn  Expr=u(4)*100*sqrt(abs((u(2)*u(3)+!u(2)*u(1))*0.000001/(u(5))))
  Valve plug diameter in [mm] : Constant  Value=50
  Valve recovery coefficient Km=f(X) : Lookup  InputValues=[0 10 20 30 40 50 60 70 80 90 99 100]  Table=[1.00 0.95 0.90 0.85 0.785 0.725 0.67 0.61 0.555 0.5 0.45 0.40]  SaturateOnIntegerOverflow=on
  Vena contracta pressure [Pa] : Fcn  Expr=u(3)-u(1)/u(2)
  Vena contracta force Fvc [N] : Fcn  Expr=(u(1)-u(2))*pi*u(3)*u(3)/4000000
  Water vapor pv pressure in [Pa] : Fcn  Expr=exp(ln(10)*((-2141/(u+273.15)+10.7167)))
  rc*pv : Product  SaturateOnIntegerOverflow=on  RndMeth=Zero  InputSameDT=on  OutDataTypeStr=Inherit: Same as first input
  water specific gravity : Subsystem
  Fvc[N] : Outport
  Fv[t/h] : Outport  Port=2
  wires:
  Kv(X)/1 -> Mux3/4
  Errossion fault  f3 X negative offset/1(Xf[%]) -> Scalling factor/1, Equipercentage rated flow coefficient/1(X[%])
  X[%]/1 -> Sedimentation fault  f2 X positive offset/1(X[%])
  "Errosion fault  f3 gaining Kvr "/1(Kvrf[%]) -> Internal leakage fault  f6 additive fault/1(Kvr[%])
  f3<0,1>/1 -> "Errosion fault  f3 gaining Kvr "/2(f3<0,1>), Errossion fault  f3 X negative offset/2(f3<0,1>)
  Sedimentation fault  f2 Kvr lowering/1(Kvrf[%]) -> "Errosion fault  f3 gaining Kvr "/1(Kvr[%])
  f2<0,1>/1 -> Sedimentation fault  f2 Kvr lowering/2(f2<0,1>), Sedimentation fault  f2 X positive offset/2(f2<0,1>)
  Equipercentage rated flow coefficient/1(Kvr[%]) -> Sedimentation fault  f2 Kvr lowering/1(Kvr[%])
  Sedimentation fault  f2 X positive offset/1(Xf[%]) -> Errossion fault  f3 X negative offset/1(X[%])
  Internal leakage fault  f6 additive fault/1(Kvrf[%]) -> Kv(X)/1
  " Valve Kv n=5"/1 -> Kv(X)/2
  f6<0,1>/1 -> Internal leakage fault  f6 additive fault/2(f6<0,1>)
  Mux3/1 -> Square root flow law Qv[m^3/h]/1
  Vena contracta force Fvc [N]/1 -> Fvc[N]/1
  Qv*ro/1 -> Fv[t/h]/1
  Scalling factor [t/kg]/1 -> Qv*ro/2
  Square root flow law Qv[m^3/h]/1 -> Qv*ro/1
  Pressure limiter/1 -> Mux3/2
  Mux7/1 -> Vena contracta force Fvc [N]/1
  Water vapor pv pressure in [Pa]/1 -> P1>pv/2, rc*pv/2
  Vena contracta pressure [Pa]/1 -> Mux7/2
  P1>pv/1 -> Mux7/1, water specific gravity/1(P[Pa]), Mux6/3, P1-P2/1, "Critical pressure ratio for the water rc=f(pv[Pa]) "/1, P1-rc*pv [Pa]/1
  P1[Pa]/1 -> P1>pv/1
  Valve plug diameter in [mm]/1 -> Mux7/3
  Valve recovery coefficient Km=f(X)/1 -> Mux6/2, Km(P1-rc*pv)/2
  water specific gravity/1(ro[kg/m^3]) -> Scalling factor [t/kg]/1, Mux3/5
  Scalling factor/1 -> Valve recovery coefficient Km=f(X)/1
  T1[C]/1 -> water specific gravity/2(T[C]), Water vapor pv pressure in [Pa]/1
  Saturation >0/1 -> Mux3/1, Pressure limiter/1
  rc*pv/1 -> P1-rc*pv [Pa]/2
  P1-rc*pv [Pa]/1 -> Km(P1-rc*pv)/1
  Km(P1-rc*pv)/1 -> Saturation >0/1
  "Critical pressure ratio for the water rc=f(pv[Pa]) "/1 -> rc*pv/1
  P2[Pa]/1 -> P1-P2/2
  P1-P2/1 -> Mux3/3, Pressure limiter/2, Mux6/1
  Mux6/1 -> Vena contracta pressure [Pa]/1

== system DABLib/DABLibUtil/CoreAct+/Unexpected pressure change across the valve f17 ==
  note: Fault  f17
      | Unexpected pressure drop accross the valve
  P1[Pa] : Inport
  P2[Pa] : Inport  Port=2
  f17<-1,1> : Inport  Port=3
  " " : Fcn  Expr=u(4)*(1-u(3)*abs(u(2)))
  " 1" : Fcn  Expr=u(1)*(1-!u(3)*abs(u(2)))
  "0..4MPa " : Saturate  UpperLimit=4000000  LowerLimit=0
  0..4MPa 1 : Saturate  UpperLimit=4000000  LowerLimit=0
  Environment pressure [kPa]3 : Constant  Value=0
  "Fault streght saturation " : Saturate  UpperLimit=1.0  LowerLimit=-1.0
  Mux4 : Mux
  Relational Operator1 : RelationalOperator  Operator=>  RndMeth=Nearest  InputSameDT=on
  P1f[Pa] : Outport
  P2f[Pa] : Outport  Port=2
  wires:
  P2[Pa]/1 -> Mux4/4
  Relational Operator1/1 -> Mux4/3
  "Fault streght saturation "/1 -> Mux4/2, Relational Operator1/1
  Environment pressure [kPa]3/1 -> Relational Operator1/2
  f17<-1,1>/1 -> "Fault streght saturation "/1
  P1[Pa]/1 -> Mux4/1
  Mux4/1 -> " 1"/1, " "/1
  0..4MPa 1/1 -> P1f[Pa]/1
  " 1"/1 -> 0..4MPa 1/1
  " "/1 -> "0..4MPa "/1
  "0..4MPa "/1 -> P2f[Pa]/1

== system DABLib/DABLibUtil/Det or Iso/Subsystem ==
  t_from : Inport
  fs : Inport  Port=2
  Enable : EnablePort
  Trigger : TriggerPort  VariantControl=Variant
  Digital Clock : DigitalClock  SampleTime=-1
  Sum : Sum  Inputs=+-  SaturateOnIntegerOverflow=on  InputSameDT=on  OutDataTypeStr=Inherit: Same as first input
  Switch : Switch  SaturateOnIntegerOverflow=on  InputSameDT=on
  Switch1 : Switch  SaturateOnIntegerOverflow=on  InputSameDT=on
  t_dt : Outport  InitialOutput=-1
  fs_d : Outport  Port=2  InitialOutput=-1
  wires:
  Digital Clock/1 -> Sum/1
  Switch1/1 -> fs_d/1
  fs/1 -> Switch1/1
  Switch/1 -> t_dt/1
  Sum/1 -> Switch/1
  t_from/1 -> Switch1/3, Switch1/2, Switch/3, Switch/2, Sum/2

== system DABLib/DABLibUtil/Det or Iso/Subsystem1 ==
  t_to : Inport
  Enable : EnablePort
  Trigger : TriggerPort  TriggerType=falling  VariantControl=Variant
  Digital Clock : DigitalClock  SampleTime=-1
  Sum1 : Sum  Inputs=-+  SaturateOnIntegerOverflow=on  InputSameDT=on  OutDataTypeStr=Inherit: Same as first input
  Switch2 : Switch  SaturateOnIntegerOverflow=on  InputSameDT=on
  t_drt : Outport  InitialOutput=-1
  wires:
  Digital Clock/1 -> Sum1/2
  Switch2/1 -> t_drt/1
  t_to/1 -> Switch2/3, Switch2/2, Sum1/1
  Sum1/1 -> Switch2/1

== system DABLib/DABLibUtil/Det or Iso/subsystem ==
  t_on : Inport
  t_from : Inport  Port=2
  t_to : Inport  Port=3
  t_hor : Inport  Port=4
  td : Inport  Port=5
  fd : Inport  Port=6
  Enable : EnablePort
  0 Proof Division with -1 correction : DABLib/DABLibUtil/0 Proof Division with -1 correction
  "0 Proof Division with -1 correction " : DABLib/DABLibUtil/0 Proof Division with -1 correction
  "0, t-t1>0, t2 or 0" : DABLib/DABLibUtil/0, t-t1>0, t2 or 0
  "0, t-t1>0, t2 or 0 " : DABLib/DABLibUtil/0, t-t1>0, t2 or 0
  "0, t-t1>0, t2 or 0  " : DABLib/DABLibUtil/0, t-t1>0, t2 or 0
  Sum : Sum  Inputs=2  SaturateOnIntegerOverflow=on  InputSameDT=on  OutDataTypeStr=Inherit: Same as first input
  r_td : Outport  InitialOutput=-1
  r_fd : Outport  Port=2  InitialOutput=-1
  wires:
  "0, t-t1>0, t2 or 0  "/1 -> "0 Proof Division with -1 correction "/1
  "0, t-t1>0, t2 or 0 "/1 -> Sum/2
  "0, t-t1>0, t2 or 0"/1 -> Sum/1
  Sum/1 -> 0 Proof Division with -1 correction/1
  0 Proof Division with -1 correction/1 -> r_fd/1
  fd/1 -> 0 Proof Division with -1 correction/2
  td/1 -> "0 Proof Division with -1 correction "/2
  "0 Proof Division with -1 correction "/1 -> r_td/1
  t_from/1 -> "0, t-t1>0, t2 or 0  "/2, "0, t-t1>0, t2 or 0 "/1
  t_to/1 -> "0, t-t1>0, t2 or 0  "/1, "0, t-t1>0, t2 or 0"/2
  t_on/1 -> "0, t-t1>0, t2 or 0 "/2
  t_hor/1 -> "0, t-t1>0, t2 or 0"/1

== system DABLib/DABLibUtil/Tranducer/Sensor fault  ==
  note: Flow sensor fault
  X[%] : Inport
  fs<-1,1>] : Inport  Port=2
  " " : Fcn  Expr=u(1)*(1-u(2)*u(3))
  Fault range in [%] <0..1> : Constant  Value=1.00
  "Fault streght saturation -100..100% " : Saturate  UpperLimit=1.0  LowerLimit=-1.0
  Mux4 : Mux  Inputs=3
  "Sensor range 0..1 " : Saturate  UpperLimit=1  LowerLimit=0
  Sensor range 0..100% : Saturate  UpperLimit=1.00  LowerLimit=0
  Xf[%] : Outport
  wires:
  Sensor range 0..100%/1 -> Xf[%]/1
  " "/1 -> Sensor range 0..100%/1
  "Sensor range 0..1 "/1 -> Mux4/1
  X[%]/1 -> "Sensor range 0..1 "/1
  Fault range in [%] <0..1>/1 -> Mux4/2
  "Fault streght saturation -100..100% "/1 -> Mux4/3
  fs<-1,1>]/1 -> "Fault streght saturation -100..100% "/1
  Mux4/1 -> " "/1

== system DABLib/PICalc/Zones Selection/Stop-watch 1st ==
  TR st : Inport
  Enable : EnablePort
  BZ-Fault Free 2 : Logic
  BZ-Fault Free 3 : Logic  Operator=NOT  Inputs=1
  Memory : Memory
  Stop-watch : Subsystem
  t(k) : Outport
  wires:
  Stop-watch/1(t(k)) -> t(k)/1
  TR st/1 -> BZ-Fault Free 2/1
  Memory/1 -> BZ-Fault Free 3/1
  BZ-Fault Free 3/1 -> BZ-Fault Free 2/2
  BZ-Fault Free 2/1 -> Stop-watch/Trigger
  Stop-watch/2(TR) -> Memory/1

== system DABLib/PICalc/Zones Selection/Stop-watch last ==
  Enable : EnablePort
  Trigger : TriggerPort  TriggerType=falling  VariantControl=Variant
  Digital Clock : DigitalClock  SampleTime=-1
  t(k) : Outport  InitialOutput=-1
  wires:
  Digital Clock/1 -> t(k)/1

== system DABLib/DABLibUtil/CoreAct/  E//P transducer/Electro-pneumatic transducer  fault f12 ==
  note: Fault  f12
      | Electro-pneumatic transducer fault
  I[%] : Inport
  f12<-1,1>] : Inport  Port=2
  " " : Fcn  Expr=u(1)*(1-u(2)*u(3))
  Fault range <0..1> : Constant  Value=1.0
  "Fault streght saturation -100..100% " : Saturate  UpperLimit=1.0  LowerLimit=-1.0
  "If saturation -100..100% " : Saturate  UpperLimit=1.0  LowerLimit=-1.0
  Mux4 : Mux  Inputs=3
  If[%] : Outport
  wires:
  "If saturation -100..100% "/1 -> If[%]/1
  " "/1 -> "If saturation -100..100% "/1
  Fault range <0..1>/1 -> Mux4/2
  "Fault streght saturation -100..100% "/1 -> Mux4/3
  f12<-1,1>]/1 -> "Fault streght saturation -100..100% "/1
  I[%]/1 -> Mux4/1
  Mux4/1 -> " "/1

== system DABLib/DABLibUtil/CoreAct/CVP//Ps converter/Diaphragm perforation fault f10 ==
  note: try from 0.3
  note: Fault  9
      | Servo-motor's housing or terminals tightness
      | Fault 10
      | Diaphragm perforation fault
  f9<0,1> : Inport
  f10<0,1> : Inport  Port=2
  Ps[Pa] : Inport  Port=3
  " " : Fcn  Expr=u(1)*u(2)+u(2)*u(3)
  Fault range <0..1> : Constant  Value=0.1
  "Fault streght saturation 0..100% " : Saturate  UpperLimit=1  LowerLimit=0
  Fault streght saturation 0..100% 1 : Saturate  UpperLimit=1  LowerLimit=0
  Mux4 : Mux  Inputs=3
  P13 : Product  SaturateOnIntegerOverflow=on  RndMeth=Zero  InputSameDT=on  OutDataTypeStr=Inherit: Same as first input
  leakage flow : Fcn  Expr=sqrt(abs(u))*2e-6
  mdotl[kg/s] : Outport
  wires:
  P13/1 -> mdotl[kg/s]/1
  leakage flow/1 -> P13/2
  Ps[Pa]/1 -> leakage flow/1
  " "/1 -> P13/1
  Fault streght saturation 0..100% 1/1 -> Mux4/1
  f9<0,1>/1 -> Fault streght saturation 0..100% 1/1
  "Fault streght saturation 0..100% "/1 -> Mux4/3
  Mux4/1 -> " "/1
  Fault range <0..1>/1 -> Mux4/2
  f10<0,1>/1 -> "Fault streght saturation 0..100% "/1

== system DABLib/DABLibUtil/CoreAct/Positioner feedback/Positioner feedback fault f15 ==
  note: dead band in [m]
  note: Fault  f15
      | Positioner spring  fault
      | Positioner feedback fault
  Xn[m] : Inport
  f15<0,1> : Inport  Port=2
  " " : Fcn  Expr=u(1)*u(2)*u(3)
  Fault range in [%] <0..1> : Constant  Value=1.0
  "Fault streght saturation " : Saturate  UpperLimit=1.0  LowerLimit=0
  Mux4 : Mux  Inputs=3
  Df[m] : Outport
  wires:
  Fault range in [%] <0..1>/1 -> Mux4/2
  "Fault streght saturation "/1 -> Mux4/3
  " "/1 -> Df[m]/1
  f15<0,1>/1 -> "Fault streght saturation "/1
  Xn[m]/1 -> Mux4/1
  Mux4/1 -> " "/1

== system DABLib/DABLibUtil/CoreAct/Positioner feedback/WUT Backlash ==
  signal : Inport
  dead band : Inport  Port=2
  Hysteresis : Subsystem
  Memory1 : Memory
  WUT direction decoder : Subsystem
  output : Outport
  wires:
  Hysteresis/1(hysta) -> Memory1/1, output/1
  Memory1/1 -> Hysteresis/4(history)
  dead band/1 -> Hysteresis/3(h_band)
  WUT direction decoder/1(direction) -> Hysteresis/2(x_dir)
  signal/1 -> Hysteresis/1(x), WUT direction decoder/1("signal ")

== system DABLib/DABLibUtil/CoreAct/Ps//X transducer Pneumatic servo-motor/Dynamic force ==
  Fd'A [N] : Inport
  X<=Lb : Inport  Port=2
  X>=Hb : Inport  Port=3
  "Dynamic force F is equal to zero if Lower Bound is reached and  Fd'A<=0 or if Higher Bound is reached and Fd'A>=0    " : Fcn  Expr=u[1]*((1-u[2]*u[3])*(1-(1-u[2])*u[4]))
  Logical Operator : Logic  Operator=OR
  Mux1 : Mux
  Operator logiczny3 : RelationalOperator  Operator=<=  RndMeth=Nearest  InputSameDT=on
  zero : Constant  Value=0
  F [N] : Outport
  V reset : Outport  Port=2
  wires:
  zero/1 -> Operator logiczny3/2
  Operator logiczny3/1 -> Mux1/2
  Fd'A [N]/1 -> Mux1/1, Operator logiczny3/1
  Mux1/1 -> "Dynamic force F is equal to zero if Lower Bound is reached and  Fd'A<=0 or if Higher Bound is reached and Fd'A>=0    "/1
  "Dynamic force F is equal to zero if Lower Bound is reached and  Fd'A<=0 or if Higher Bound is reached and Fd'A>=0    "/1 -> F [N]/1
  X>=Hb/1 -> Mux1/4, Logical Operator/1
  X<=Lb/1 -> Mux1/3, Logical Operator/2
  Logical Operator/1 -> V reset/1

== system DABLib/DABLibUtil/CoreAct/Ps//X transducer Pneumatic servo-motor/Friction faultf4 ==
  note: Fault  f4
      | Increased friction fault
  Hb[m] : Inport
  f4<-1,1> : Inport  Port=2
  " " : Fcn  Expr=u(1)*(u(2)+u(3))
  "Deadband 0..0.0381m " : Saturate  UpperLimit=0.0381  LowerLimit=0
  "Fault streght saturation -100..100% " : Saturate  UpperLimit=1.0  LowerLimit=-1.0
  Higher bound 0..0.0381 : Saturate  UpperLimit=0.0381  LowerLimit=0
  Mux4 : Mux  Inputs=3
  Nominal hysteresis [%] : Constant  Value=0.01
  Dbf[m] : Outport
  wires:
  " "/1 -> "Deadband 0..0.0381m "/1
  Mux4/1 -> " "/1
  "Deadband 0..0.0381m "/1 -> Dbf[m]/1
  Higher bound 0..0.0381/1 -> Mux4/1
  Hb[m]/1 -> Higher bound 0..0.0381/1
  Nominal hysteresis [%]/1 -> Mux4/2
  "Fault streght saturation -100..100% "/1 -> Mux4/3
  f4<-1,1>/1 -> "Fault streght saturation -100..100% "/1

== system DABLib/DABLibUtil/CoreAct/Ps//X transducer Pneumatic servo-motor/Programable saturation ==
  note: Programmable saturation
  Hb[m] : Inport
  X[m] : Inport  Port=2
  "Displacement lower limit 0..inf " : Saturate  UpperLimit=inf  LowerLimit=0
  Mux8 : Mux  Inputs=3
  Programmable saturation : Fcn  Expr=u(1)*u(2)+u(3)*!u(2)
  Relational Operator : RelationalOperator  Operator=<=  RndMeth=Nearest  InputSameDT=on
  Xl[m] : Outport
  1 if Hb<=X : Outport  Port=2
  wires:
  Programmable saturation/1 -> Xl[m]/1
  "Displacement lower limit 0..inf "/1 -> Relational Operator/2, Mux8/3
  X[m]/1 -> "Displacement lower limit 0..inf "/1
  Hb[m]/1 -> Relational Operator/1, Mux8/1
  Mux8/1 -> Programmable saturation/1
  Relational Operator/1 -> Mux8/2, 1 if Hb<=X/1

== system DABLib/DABLibUtil/CoreAct/Ps//X transducer Pneumatic servo-motor/Sedimentation fault f2 ==
  note: Fault  f2
      | Valve plug or valve seat
      | sedimentation fault
  Hb[m] : Inport
  f2<0,1> : Inport  Port=2
  " " : Fcn  Expr=u(1)*(1-u(2)*u(3))
  "Fault streght saturation 0..100% " : Saturate  UpperLimit=1.0  LowerLimit=-1.0
  Higher bound limit 0..0.0381m : Saturate  UpperLimit=0.0381  LowerLimit=0
  "Higher bound limit 0..0.0381m " : Saturate  UpperLimit=0.0381  LowerLimit=0
  Mux4 : Mux  Inputs=3
  Relative sedimentation span : Constant  Value=0.2
  Hbf[m] : Outport
  wires:
  Relative sedimentation span/1 -> Mux4/2
  "Fault streght saturation 0..100% "/1 -> Mux4/3
  Higher bound limit 0..0.0381m/1 -> Mux4/1
  Hb[m]/1 -> Higher bound limit 0..0.0381m/1
  " "/1 -> "Higher bound limit 0..0.0381m "/1
  Mux4/1 -> " "/1
  "Higher bound limit 0..0.0381m "/1 -> Hbf[m]/1
  f2<0,1>/1 -> "Fault streght saturation 0..100% "/1

== system DABLib/DABLibUtil/CoreAct/Ps//X transducer Pneumatic servo-motor/Servo-motors' spring fault f11 ==
  note: Fault  f11
      | Servo-motor's spring fault
  f11<0,1> : Inport
  Fs[N] : Inport  Port=2
  " " : Fcn  Expr=u(1)*(1-u(2)*u(3))
  Fault range in [%] <0..1> : Constant  Value=1.0
  "Fault streght saturation " : Saturate  UpperLimit=1.0  LowerLimit=0
  Mux4 : Mux  Inputs=3
  Fsf[N] : Outport
  wires:
  Fault range in [%] <0..1>/1 -> Mux4/2
  "Fault streght saturation "/1 -> Mux4/3
  " "/1 -> Fsf[N]/1
  f11<0,1>/1 -> "Fault streght saturation "/1
  Fs[N]/1 -> Mux4/1
  Mux4/1 -> " "/1
